simulink model "hw7_6"  (R2022a)
settings: Solver=VariableStepAuto  StartTime=0.0  StopTime=10.0  RelTol=1e-3
settings Model: Creator=prafu  LastModifiedBy=prafu

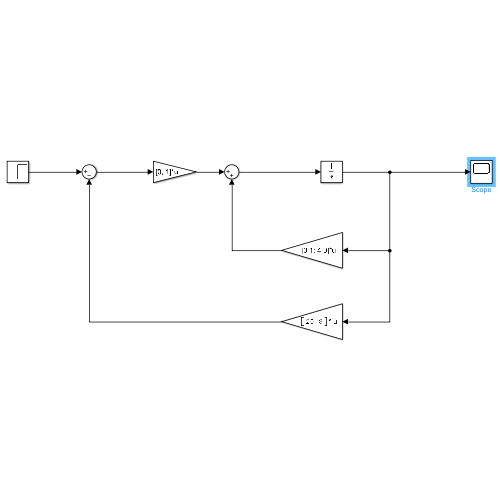
[thumbnail: Simulink's stored preview of the top-level diagram]
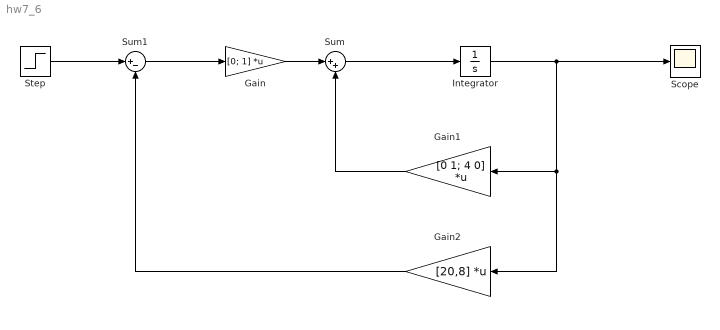
== system hw7_6 ==
  Gain : Gain  Gain=[0; 1]  Multiplication=Matrix(K*u)
  Gain1 : Gain  Gain=[0 1; 4 0]  Multiplication=Matrix(K*u)
  Gain2 : Gain  Gain=[20,8]  Multiplication=Matrix(K*u)
  Integrator : Integrator  InitialCondition=[2;1]
  Scope : Scope
  Step : Step  SampleTime=0
  Sum : Sum  Inputs=|++
  Sum1 : Sum  Inputs=|+-
  wires:
  Gain/1 -> Sum/1
  Sum/1 -> Integrator/1
  Integrator/1 -> Gain2/1, Gain1/1, Scope/1
  Gain1/1 -> Sum/2
  Gain2/1 -> Sum1/2
  Step/1 -> Sum1/1
  Sum1/1 -> Gain/1
